simulink model "CLF_CBF_QP_Controller"  (R2026a)
settings: Solver=VariableStepAuto  StopTime=65  AbsTol=1e-4
PostLoadFcn:
  | waypoints = [0 0; 4 2; 3 7; -3 6];
  | target_vel = 0.5;
  | lookahead_d = 2;
  | max_yaw_rate = 1;
values from neighbouring files (symbols this model uses):
  m = max(2, ceil(Lseg/ds))    [Trajectory.m]    (also in plot_nmpc_result.m = NaN)
  s = [0; cumsum(hypot(diff(xs),diff(ys)))]    [Trajectory.m]    (also in plot_parking_mpc.m = evalin('base',name); plot_result.m = out.(names{k}))
  trajMatrix = [tvec, xd, yd, thd, vd, wd]    [Trajectory.m]    (also in plot_parking_mpc.m = evalin('base','trajMatrix'); plot_result.m = evalin('base','trajMatrix'))
undefined symbols (not defined in the file or in its folder): X, Y, Z
libraries: sm_lib x104, nesl_utility x11, slpidlib x1, simulink x1
(part 3 of 3)

== system CLF_CBF_QP_Controller/Robot/Wheel L/left_wheel ==
  Inertia : sm_lib/Body Elements/Inertia  InertiaType=Custom  Mass=0.1  MassUnits=kg  CenterOfMass=[0, 0, 0]  CenterOfMassUnits=m  MomentsOfInertia=[1, 1, 1]*0.01  MomentsOfInertiaUnits=kg*m^2  ProductsOfInertia=[0, 0, 0]  ProductsOfInertiaUnits=kg*m^2  GraphicType=None  MarkerShape=Inertia  MarkerSize=20  GraphicVisPropType=SimpleVisualProperties  GraphicDiffuseColor=[0.5 0.5 0.5]  GraphicOpacity=1.0  GraphicSpecularColor=[0.5 0.5 0.5 1.0]  GraphicAmbientColor=[0.15 0.15 0.15 1.0]  GraphicEmissiveColor=[0.0 0.0 0.0 1.0]  GraphicShininess=75
  InertiaOriginTransform : sm_lib/Frames and Transforms/Rigid Transform  RotationMethod=RotationSequence  FollAlignAxisA=+X  BaseAlignAxisA=+Y  FollAlignAxisB=+Y  BaseAlignAxisB=+Z  RotationStandardAxis=+Z  RotationAngle=0.0  RotationAngleUnits=deg  RotationArbitraryAxis=[0 0 1]  RotationSequenceAxes=BaseAxes  RotationSequence=XYZ  RotationSequenceAngles=[0, 0, 0]  RotationSequenceAnglesUnits=rad  RotationMatrix=[1 0 0; 0 1 0; 0 0 1]  Quaternion=[1 0 0 0]  TranslationMethod=Cartesian  TranslationCartesianOffset=[0, 0, 0]  TranslationCartesianOffsetUnits=m  TranslationStandardAxis=+Z  TranslationStandardOffset=0  TranslationStandardOffsetUnits=m  TranslationROffset=0  TranslationROffsetUnits=m  TranslationThetaOffset=0  TranslationThetaOffsetUnits=deg  TranslationZOffset=0  TranslationZOffsetUnits=m
  ReferenceFrame : sm_lib/Frames and Transforms/Reference Frame
  Spherical Solid For Contact : sm_lib/Body Elements/Spherical Solid  SphereRadius=0.0925  SphereRadiusUnits=m  ExportEntireGeometry=on  InertiaType=Custom  BasedOnType=Density  Density=1000  DensityUnits=kg/m^3  Mass=0  MassUnits=kg  CenterOfMass=[0 0 0]  CenterOfMassUnits=m  MomentsOfInertia=[0 0 0]  MomentsOfInertiaUnits=kg*m^2  ProductsOfInertia=[0 0 0]  ProductsOfInertiaUnits=kg*m^2  GraphicType=FromGeometry  MarkerShape=Sphere  MarkerSize=10  GraphicVisPropType=SimpleVisualProperties  GraphicDiffuseColor=clr_contact_sphere  GraphicOpacity=opc_contact_sphere  GraphicSpecularColor=[0.5 0.5 0.5 1.0]  GraphicAmbientColor=[0.15 0.15 0.15 1.0]  GraphicEmissiveColor=[0.0 0.0 0.0 1.0]  GraphicShininess=75  DoExposeReferenceFrame=on  SerializedFrames=<Frames/>
  Visual : sm_lib/Body Elements/File Solid  ExtGeomFileName=amr3dx_left_wheel.stl  UnitType=Custom  ExtGeomFileUnits=m  StepReaderType=HEX  ExportConvexHullGeometry=off  InertiaType=Custom  BasedOnType=DensityFromFile  Density=1000  DensityUnits=kg/m^3  Mass=0  MassUnits=kg  CenterOfMass=[0, 0, 0]  CenterOfMassUnits=m  MomentsOfInertia=[0, 0, 0]  MomentsOfInertiaUnits=kg*m^2  ProductsOfInertia=[0, 0, 0]  ProductsOfInertiaUnits=kg*m^2  GraphicType=FromGeometry  MarkerShape=Sphere  MarkerSize=10  GraphicVisPropType=SimpleVisualProperties  GraphicDiffuseColor=[0.117, 0.117, 0.117]  GraphicOpacity=1  GraphicSpecularColor=[0.5 0.5 0.5 1.0]  GraphicAmbientColor=[0.15 0.15 0.15 1.0]  GraphicEmissiveColor=[0.0 0.0 0.0 1.0]  GraphicShininess=75  DoExposeReferenceFrame=on  SerializedFrames=<Frames/>
  VisualOriginTransform : sm_lib/Frames and Transforms/Rigid Transform  RotationMethod=RotationSequence  FollAlignAxisA=+X  BaseAlignAxisA=+Y  FollAlignAxisB=+Y  BaseAlignAxisB=+Z  RotationStandardAxis=+Z  RotationAngle=0.0  RotationAngleUnits=deg  RotationArbitraryAxis=[0 0 1]  RotationSequenceAxes=BaseAxes  RotationSequence=XYZ  RotationSequenceAngles=[0, 0, 0]  RotationSequenceAnglesUnits=rad  RotationMatrix=[1 0 0; 0 1 0; 0 0 1]  Quaternion=[1 0 0 0]  TranslationMethod=Cartesian  TranslationCartesianOffset=[0, 0, 0]  TranslationCartesianOffsetUnits=m  TranslationStandardAxis=+Z  TranslationStandardOffset=0  TranslationStandardOffsetUnits=m  TranslationROffset=0  TranslationROffsetUnits=m  TranslationThetaOffset=0  TranslationThetaOffsetUnits=deg  TranslationZOffset=0  TranslationZOffsetUnits=m
  F : PMIOPort  Side=Left
  G : PMIOPort  Port=2  Side=Left
  connections:
  Inertia/RConn1 -- InertiaOriginTransform/RConn1
  ReferenceFrame/RConn1 -- F/RConn1 -- InertiaOriginTransform/LConn1 -- VisualOriginTransform/LConn1
  G/RConn1 -- Spherical Solid For Contact/LConn1
  Visual/RConn1 -- Spherical Solid For Contact/RConn1 -- VisualOriginTransform/RConn1

== system CLF_CBF_QP_Controller/Robot/WheelR/right_hub ==
  ReferenceFrame : sm_lib/Frames and Transforms/Reference Frame
  Visual : sm_lib/Body Elements/File Solid  ExtGeomFileName=amr3dx_right_hubcap.stl  UnitType=Custom  ExtGeomFileUnits=m  StepReaderType=HEX  ExportConvexHullGeometry=off  InertiaType=Custom  BasedOnType=DensityFromFile  Density=1000  DensityUnits=kg/m^3  Mass=0  MassUnits=kg  CenterOfMass=[0, 0, 0]  CenterOfMassUnits=m  MomentsOfInertia=[0, 0, 0]  MomentsOfInertiaUnits=kg*m^2  ProductsOfInertia=[0, 0, 0]  ProductsOfInertiaUnits=kg*m^2  GraphicType=FromGeometry  MarkerShape=Sphere  MarkerSize=10  GraphicVisPropType=SimpleVisualProperties  GraphicDiffuseColor=[1, 0.8110000000000001, 0.151]  GraphicOpacity=1  GraphicSpecularColor=[0.5 0.5 0.5 1.0]  GraphicAmbientColor=[0.15 0.15 0.15 1.0]  GraphicEmissiveColor=[0.0 0.0 0.0 1.0]  GraphicShininess=75  DoExposeReferenceFrame=on  SerializedFrames=<Frames/>
  VisualOriginTransform : sm_lib/Frames and Transforms/Rigid Transform  RotationMethod=RotationSequence  FollAlignAxisA=+X  BaseAlignAxisA=+Y  FollAlignAxisB=+Y  BaseAlignAxisB=+Z  RotationStandardAxis=+Z  RotationAngle=0.0  RotationAngleUnits=deg  RotationArbitraryAxis=[0 0 1]  RotationSequenceAxes=BaseAxes  RotationSequence=XYZ  RotationSequenceAngles=[0, 0, 0]  RotationSequenceAnglesUnits=rad  RotationMatrix=[1 0 0; 0 1 0; 0 0 1]  Quaternion=[1 0 0 0]  TranslationMethod=Cartesian  TranslationCartesianOffset=[0, 0, 0]  TranslationCartesianOffsetUnits=m  TranslationStandardAxis=+Z  TranslationStandardOffset=0  TranslationStandardOffsetUnits=m  TranslationROffset=0  TranslationROffsetUnits=m  TranslationThetaOffset=0  TranslationThetaOffsetUnits=deg  TranslationZOffset=0  TranslationZOffsetUnits=m
  right_hub_joint_AxisInvTransform : sm_lib/Frames and Transforms/Rigid Transform  RotationMethod=ArbitraryAxis  FollAlignAxisA=+X  BaseAlignAxisA=+Y  FollAlignAxisB=+Y  BaseAlignAxisB=+Z  RotationStandardAxis=+Z  RotationAngle=1.570796326794897  RotationAngleUnits=rad  RotationArbitraryAxis=[-1, 0, 0]  RotationSequenceAxes=FollowerAxes  RotationSequence=XYX  RotationSequenceAngles=[0 0 0]  RotationSequenceAnglesUnits=deg  RotationMatrix=[1 0 0; 0 1 0; 0 0 1]  Quaternion=[1 0 0 0]  TranslationMethod=Cartesian  TranslationCartesianOffset=[0, 0, 0]  TranslationCartesianOffsetUnits=m  TranslationStandardAxis=+Z  TranslationStandardOffset=0  TranslationStandardOffsetUnits=m  TranslationROffset=0  TranslationROffsetUnits=m  TranslationThetaOffset=0  TranslationThetaOffsetUnits=deg  TranslationZOffset=0  TranslationZOffsetUnits=m
  right_wheel_joint_OriginTransform : sm_lib/Frames and Transforms/Rigid Transform  RotationMethod=RotationSequence  FollAlignAxisA=+X  BaseAlignAxisA=+Y  FollAlignAxisB=+Y  BaseAlignAxisB=+Z  RotationStandardAxis=+Z  RotationAngle=0.0  RotationAngleUnits=deg  RotationArbitraryAxis=[0 0 1]  RotationSequenceAxes=BaseAxes  RotationSequence=XYZ  RotationSequenceAngles=[0, 0, 0]  RotationSequenceAnglesUnits=rad  RotationMatrix=[1 0 0; 0 1 0; 0 0 1]  Quaternion=[1 0 0 0]  TranslationMethod=Cartesian  TranslationCartesianOffset=[0, 0, 0]  TranslationCartesianOffsetUnits=m  TranslationStandardAxis=+Z  TranslationStandardOffset=0  TranslationStandardOffsetUnits=m  TranslationROffset=0  TranslationROffsetUnits=m  TranslationThetaOffset=0  TranslationThetaOffsetUnits=deg  TranslationZOffset=0  TranslationZOffsetUnits=m
  F : PMIOPort  Side=Left
  F1 : PMIOPort  Port=2  Side=Right
  connections:
  ReferenceFrame/RConn1 -- VisualOriginTransform/LConn1 -- right_hub_joint_AxisInvTransform/LConn1 -- right_wheel_joint_OriginTransform/LConn1
  Visual/RConn1 -- VisualOriginTransform/RConn1
  right_hub_joint_AxisInvTransform/RConn1 -- F/RConn1
  right_wheel_joint_OriginTransform/RConn1 -- F1/RConn1

== system CLF_CBF_QP_Controller/Robot/WheelR/right_wheel ==
  Inertia : sm_lib/Body Elements/Inertia  InertiaType=Custom  Mass=0.1  MassUnits=kg  CenterOfMass=[0, 0, 0]  CenterOfMassUnits=m  MomentsOfInertia=[1, 1, 1]*0.01  MomentsOfInertiaUnits=kg*m^2  ProductsOfInertia=[0, 0, 0]  ProductsOfInertiaUnits=kg*m^2  GraphicType=None  MarkerShape=Inertia  MarkerSize=20  GraphicVisPropType=SimpleVisualProperties  GraphicDiffuseColor=[0.5 0.5 0.5]  GraphicOpacity=1.0  GraphicSpecularColor=[0.5 0.5 0.5 1.0]  GraphicAmbientColor=[0.15 0.15 0.15 1.0]  GraphicEmissiveColor=[0.0 0.0 0.0 1.0]  GraphicShininess=75
  InertiaOriginTransform : sm_lib/Frames and Transforms/Rigid Transform  RotationMethod=RotationSequence  FollAlignAxisA=+X  BaseAlignAxisA=+Y  FollAlignAxisB=+Y  BaseAlignAxisB=+Z  RotationStandardAxis=+Z  RotationAngle=0.0  RotationAngleUnits=deg  RotationArbitraryAxis=[0 0 1]  RotationSequenceAxes=BaseAxes  RotationSequence=XYZ  RotationSequenceAngles=[0, 0, 0]  RotationSequenceAnglesUnits=rad  RotationMatrix=[1 0 0; 0 1 0; 0 0 1]  Quaternion=[1 0 0 0]  TranslationMethod=Cartesian  TranslationCartesianOffset=[0, 0, 0]  TranslationCartesianOffsetUnits=m  TranslationStandardAxis=+Z  TranslationStandardOffset=0  TranslationStandardOffsetUnits=m  TranslationROffset=0  TranslationROffsetUnits=m  TranslationThetaOffset=0  TranslationThetaOffsetUnits=deg  TranslationZOffset=0  TranslationZOffsetUnits=m
  ReferenceFrame : sm_lib/Frames and Transforms/Reference Frame
  Spherical Solid For Contact : sm_lib/Body Elements/Spherical Solid  SphereRadius=0.0925  SphereRadiusUnits=m  ExportEntireGeometry=on  InertiaType=Custom  BasedOnType=Density  Density=1000  DensityUnits=kg/m^3  Mass=0  MassUnits=kg  CenterOfMass=[0 0 0]  CenterOfMassUnits=m  MomentsOfInertia=[0 0 0]  MomentsOfInertiaUnits=kg*m^2  ProductsOfInertia=[0 0 0]  ProductsOfInertiaUnits=kg*m^2  GraphicType=FromGeometry  MarkerShape=Sphere  MarkerSize=10  GraphicVisPropType=SimpleVisualProperties  GraphicDiffuseColor=clr_contact_sphere  GraphicOpacity=opc_contact_sphere  GraphicSpecularColor=[0.5 0.5 0.5 1.0]  GraphicAmbientColor=[0.15 0.15 0.15 1.0]  GraphicEmissiveColor=[0.0 0.0 0.0 1.0]  GraphicShininess=75  DoExposeReferenceFrame=on  SerializedFrames=<Frames/>
  Visual : sm_lib/Body Elements/File Solid  ExtGeomFileName=amr3dx_right_wheel.stl  UnitType=Custom  ExtGeomFileUnits=m  StepReaderType=HEX  ExportConvexHullGeometry=off  InertiaType=Custom  BasedOnType=DensityFromFile  Density=1000  DensityUnits=kg/m^3  Mass=0  MassUnits=kg  CenterOfMass=[0, 0, 0]  CenterOfMassUnits=m  MomentsOfInertia=[0, 0, 0]  MomentsOfInertiaUnits=kg*m^2  ProductsOfInertia=[0, 0, 0]  ProductsOfInertiaUnits=kg*m^2  GraphicType=FromGeometry  MarkerShape=Sphere  MarkerSize=10  GraphicVisPropType=SimpleVisualProperties  GraphicDiffuseColor=[0.117, 0.117, 0.117]  GraphicOpacity=1  GraphicSpecularColor=[0.5 0.5 0.5 1.0]  GraphicAmbientColor=[0.15 0.15 0.15 1.0]  GraphicEmissiveColor=[0.0 0.0 0.0 1.0]  GraphicShininess=75  DoExposeReferenceFrame=on  SerializedFrames=<Frames/>
  VisualOriginTransform : sm_lib/Frames and Transforms/Rigid Transform  RotationMethod=RotationSequence  FollAlignAxisA=+X  BaseAlignAxisA=+Y  FollAlignAxisB=+Y  BaseAlignAxisB=+Z  RotationStandardAxis=+Z  RotationAngle=0.0  RotationAngleUnits=deg  RotationArbitraryAxis=[0 0 1]  RotationSequenceAxes=BaseAxes  RotationSequence=XYZ  RotationSequenceAngles=[0, 0, 0]  RotationSequenceAnglesUnits=rad  RotationMatrix=[1 0 0; 0 1 0; 0 0 1]  Quaternion=[1 0 0 0]  TranslationMethod=Cartesian  TranslationCartesianOffset=[0, 0, 0]  TranslationCartesianOffsetUnits=m  TranslationStandardAxis=+Z  TranslationStandardOffset=0  TranslationStandardOffsetUnits=m  TranslationROffset=0  TranslationROffsetUnits=m  TranslationThetaOffset=0  TranslationThetaOffsetUnits=deg  TranslationZOffset=0  TranslationZOffsetUnits=m
  F : PMIOPort  Side=Left
  G : PMIOPort  Port=2  Side=Left
  connections:
  Inertia/RConn1 -- InertiaOriginTransform/RConn1
  ReferenceFrame/RConn1 -- F/RConn1 -- InertiaOriginTransform/LConn1 -- VisualOriginTransform/LConn1
  VisualOriginTransform/RConn1 -- Spherical Solid For Contact/RConn1 -- Visual/RConn1
  G/RConn1 -- Spherical Solid For Contact/LConn1

== matlab function CLF_CBF_QP_Controller/CLF_CBF_QP ==
  data: pose input; vCmd output; trajectory input; yawRateCmd output; V_out output; h_out output; t input; qp_status output; e_x output; e_y output; e_theta output
function [vCmd, yawRateCmd, V_out, h_out, qp_status, e_x, e_y, e_theta] = ...
          clf_cbf_qp_trajectory_controller(pose, trajectory, t)
%#codegen
% CLF-CBF-QP controller -- explicit quadprog version.
% qp_status: 0 = nominal, 1 = CBF rows active, 3 = QP infeasible (fallback used)

a = 0.50;  Kp = 0.50;  alpha = 1.2;
vMax = 1.0;  wMax = 2.5;
aLinMax = 0.5;  aRotMax = 3.0;
hThresh = 1.0;  speedFloor = 0.3;
robotRadius = 0.30;  bodyMargin = 0.05;  alphaBody = 1.0;
pClf = 1e3;                       % CLF slack penalty (p in (3.10))

obstacles = [ 3.6, 3.5, 0.30, 0.90 ;
              0.3, 6.5, 0.30, 0.90 ];

persistent vPrev wPrev tPrev opts
if isempty(vPrev)
    vPrev = 0; wPrev = 0; tPrev = t;
    opts = optimoptions('quadprog','Algorithm','active-set','Display','off');
end
dt = max(t - tPrev, 1e-3);

x = pose(1); y = pose(2); th = pose(3);

% ---- 1. Reference at time t (unchanged) ----
tt = trajectory(:,1);
tq = min(max(t, tt(1)), tt(end));
xd = interp1(tt, trajectory(:,2), tq);  yd = interp1(tt, trajectory(:,3), tq);
thd = interp1(tt, trajectory(:,4), tq); vd = interp1(tt, trajectory(:,5), tq);
wd = interp1(tt, trajectory(:,6), tq);

% ---- 2. Nominal CLF law (unchanged) ----
pt = [x + a*cos(th); y + a*sin(th)];
nObs = size(obstacles,1);
hNowAll = zeros(nObs,1);
for k = 1:nObs
    dvec = pt - obstacles(k,1:2).';
    hNowAll(k) = dvec.'*dvec - obstacles(k,4)^2;
end
speedScale = min(1, max(speedFloor, min(hNowAll)/hThresh));
vd_eff = vd*speedScale;

ptd     = [xd + a*cos(thd); yd + a*sin(thd)];
ptd_dot = vd_eff*[cos(thd); sin(thd)] + a*wd*[-sin(thd); cos(thd)];
e  = pt - ptd;
G  = [cos(th), -a*sin(th); sin(th), a*cos(th)];
mu_nom = ptd_dot - Kp*e;
u_nom  = G \ mu_nom;
V      = 0.5*(e.'*e);

% ---- 3. Assemble the QP:  min ||u - u_nom||^2 + pClf*delta^2 ----
H = [2*eye(2), zeros(2,1); zeros(1,2), 2*pClf];
f = [-2*u_nom; 0];

A = zeros(2*nObs+1, 3);  b = zeros(2*nObs+1, 1);
hVals = zeros(nObs,1);  hBodyVals = zeros(nObs,1);
heading = [cos(th); sin(th)];
row = 0;
for k = 1:nObs
    p_obs = obstacles(k,1:2).';
    % point (steering) barrier:  -n_k.'*G*u <= alpha*h_k
    d2 = (pt - p_obs).'*(pt - p_obs);
    h  = d2 - obstacles(k,4)^2;   hVals(k) = h;
    n  = 2*(pt - p_obs);
    row = row+1;  A(row,:) = [-n.'*G, 0];  b(row) = alpha*h;
    % body barrier:  -a_k*v <= alphaBody*hBody_k
    r_body_safe = obstacles(k,3) + robotRadius + bodyMargin;
    dB = [x;y] - p_obs;
    hB = dB.'*dB - r_body_safe^2;  hBodyVals(k) = hB;
    aB = 2*(dB.'*heading);
    row = row+1;  A(row,:) = [-aB, 0, 0];    b(row) = alphaBody*hB;
end
% CLF row (soft):  e.'*G*u - delta <= e.'*ptd_dot - 2*Kp*V
row = row+1;  A(row,:) = [e.'*G, -1];  b(row) = e.'*ptd_dot - 2*Kp*V;

% actuator + slew-rate bounds INSIDE the program
lb = [max(-vMax, vPrev - aLinMax*dt); max(-wMax, wPrev - aRotMax*dt); 0];
ub = [min( vMax, vPrev + aLinMax*dt); min( wMax, wPrev + aRotMax*dt); inf];

% ---- 4. Solve ----
x0 = [vPrev; wPrev; 0];          % warm start: previous command, zero slack
[z, ~, exitflag] = quadprog(H, f, A, b, [], [], lb, ub, x0, opts);
if exitflag > 0
    v = z(1);  w = z(2);
    qp_status = double(any(A(1:2*nObs,:)*z - b(1:2*nObs) > -1e-6));  % 1 if any CBF row binds
else
    % Fallback: brake within the rate limits (safe stop is feasible by construction)
    v = max(-vMax, min(vMax, vPrev - aLinMax*dt*sign(vPrev)));
    w = 0;
    qp_status = 3;
end

% ---- 5. No post-hoc stages needed: bounds were inside the QP ----
vCmd = v;  yawRateCmd = w;
vPrev = vCmd;  wPrev = yawRateCmd;  tPrev = t;

h_out = min([hVals; hBodyVals]);
V_out = V;
e_x = e(1);  e_y = e(2);
e_theta = atan2(sin(th - thd), cos(th - thd));
end

== matlab function CLF_CBF_QP_Controller/Control/Wheel Speed Commands ==
  data: xy input; vCmd input; yawRateCmd input; waypoints input; wL output; stopThreshold input; slowThreshold input; trackWidth input; wheelRadius input; wR output
function [wL, wR] = wheelSpeed(xy, vCmd, yawRateCmd, waypoints, ...
    stopThreshold, slowThreshold, ...
    trackWidth, wheelRadius)
%#codegen
% Converts body commands (vCmd, yawRateCmd) into left/right wheel speed
% references for the PD loop. Same signature as the original block, so
% no rewiring is needed.
%
% Difference vs. the original: the distance-based SLOW ramp is removed,
% because the reference trajectory already contains its own trapezoidal
% deceleration (v_d -> 0 at the end). Slowing down again near the final
% waypoint would make the robot lag behind the moving reference.
%
% The STOP clamp is kept as a safety net: once the robot is within
% stopThreshold of the final waypoint, wheel commands are forced to zero.

%#ok<*INUSD>  (slowThreshold intentionally unused)
%
% NOTE: in the new setup, the "waypoints" port is fed by trajMatrix
% (N x 6 = [t, x_d, y_d, theta_d, v_d, omega_d]), not the old N x 2
% [x y] array. The final goal position is therefore in columns 2:3 of
% the last row, not the whole row.

% Distance to final reference point (used only for the terminal stop)
goal = waypoints(end, 2:3).';
d    = norm(xy(:) - goal);

scale = 1.0;
if d < stopThreshold
    scale = 0.0;                 % arrived: hold position
end

v = scale * vCmd;
w = scale * yawRateCmd;

% Differential-drive kinematics
wL = (v - w*trackWidth/2) / wheelRadius;
wR = (v + w*trackWidth/2) / wheelRadius;
end
